simulink library "HndDriveReq"  (R2022a)
settings: Solver=VariableStepAuto  StartTime=0.0  StopTime=10.0  RelTol=1e-3
settings Model: Creator=DELL  LastModifiedBy=DELL

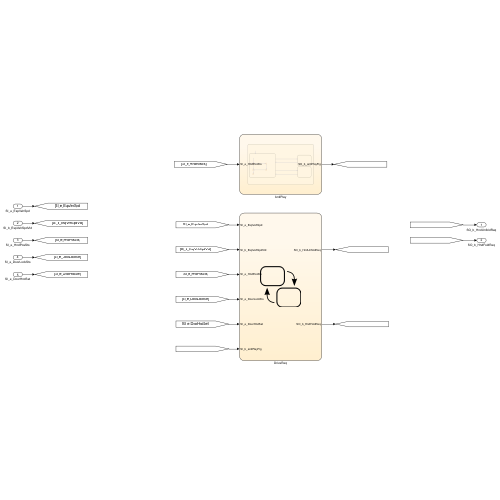
[thumbnail: Simulink's stored preview of the top-level diagram]
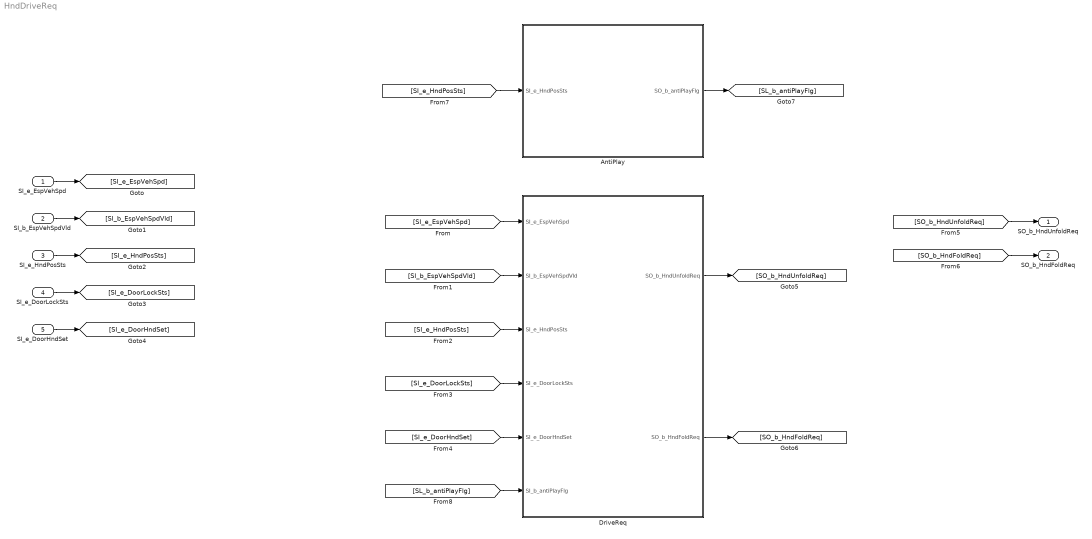
== system HndDriveReq ==
  SI_e_EspVehSpd : Inport
  SI_b_EspVehSpdVld : Inport  Port=2
  SI_e_HndPosSts : Inport  Port=3
  SI_e_DoorLockSts : Inport  Port=4
  SI_e_DoorHndSet : Inport  Port=5
  AntiPlay : Stateflow chart  TreatAsAtomicUnit=on
  DriveReq : Stateflow chart  TreatAsAtomicUnit=on
  SO_b_HndUnfoldReq : Outport
  SO_b_HndFoldReq : Outport  Port=2
  wires:
  SI_e_EspVehSpd/1 -> [SI_e_EspVehSpd]
  SI_b_EspVehSpdVld/1 -> [SI_b_EspVehSpdVld]
  SI_e_HndPosSts/1 -> [SI_e_HndPosSts]
  SI_e_DoorLockSts/1 -> [SI_e_DoorLockSts]
  SI_e_DoorHndSet/1 -> [SI_e_DoorHndSet]
  [SI_e_EspVehSpd] -> DriveReq/1(SI_e_EspVehSpd)
  [SI_b_EspVehSpdVld] -> DriveReq/2(SI_b_EspVehSpdVld)
  [SI_e_HndPosSts] -> DriveReq/3(SI_e_HndPosSts)
  [SI_e_DoorLockSts] -> DriveReq/4(SI_e_DoorLockSts)
  [SI_e_DoorHndSet] -> DriveReq/5(SI_e_DoorHndSet)
  [SO_b_HndUnfoldReq] -> SO_b_HndUnfoldReq/1
  [SO_b_HndFoldReq] -> SO_b_HndFoldReq/1
  DriveReq/1(SO_b_HndUnfoldReq) -> [SO_b_HndUnfoldReq]
  DriveReq/2(SO_b_HndFoldReq) -> [SO_b_HndFoldReq]
  [SI_e_HndPosSts] -> AntiPlay/1(SI_e_HndPosSts)
  AntiPlay/1(SO_b_antiPlayFlg) -> [SL_b_antiPlayFlg]
  [SL_b_antiPlayFlg] -> DriveReq/6(SI_b_antiPlayFlg)

== stateflow chart HndDriveReq/AntiPlay ==
  state AntiPlay
    state Count
      (default) -> (junction 4)
      Count -> (junction 4) [order 1]
      (junction 4) -> (junction 5) [order 1] : [hasChangedTo(SI_e_HndPosSts, 1) || ...
          | hasChangedTo(SI_e_HndPosSts, 0)]
      (junction 4) -> (junction 6) [order 2]
      (junction 5) -> (junction 7) : {SL_e_antiPlayCount ++}
      (junction 7) -> (junction 6)
      (junction 6) -> (junction 9)
    state TrigAndClean
      en:
      SO_b_antiPlayFlg = 1;
      SL_e_antiPlayCount = 0;
    state Clean
      en:
      SL_e_antiPlayCount = 0;
    (default) -> Count
    Count -> TrigAndClean [order 1] : [before(3000, tick) &&...
        | SL_e_antiPlayCount >= 10]
    TrigAndClean -> Count : after(18000, tick)
        | {SO_b_antiPlayFlg = 0;}
    Count -> Clean [order 2] : [after(3000, tick)]
    Clean -> Count
  data: SL_e_antiPlayCount local uint8 =0; SI_e_HndPosSts input uint8 =0; SO_b_antiPlayFlg output boolean =0

== stateflow chart HndDriveReq/DriveReq ==
  state Unfold [parallel]
    settings: executionOrder=1
    state Idle
      SO_b_HndUnfoldReq = 0;
    state NormalUnfoldReq
      en:
      SO_b_HndUnfoldReq = 1;
      on at(5, tick):
      SO_b_HndUnfoldReq = 0;
    state ExhibUnfoldReq
      en:
      SO_b_HndUnfoldReq = 1;
    state WashUnfoldReq
      en:
      SO_b_HndUnfoldReq = 1;
    (default) -> Unfold.Idle
    Unfold.Idle -> NormalUnfoldReq [order 1] : [((SI_e_EspVehSpd <= 20 && SI_b_EspVehSpdVld == 0) || ...
        | SI_b_EspVehSpdVld == 1) && ...
        | (SI_b_DoorAjar == 1 || SI_e_DoorLockSts == 1) && ...
        | SI_e_HndPosSts != 1]
    NormalUnfoldReq -> Unfold.Idle : [(SI_e_EspVehSpd > 20 && SI_b_EspVehSpdVld == 0) || ...
        | (SI_b_DoorAjar != 1 && SI_e_DoorLockSts != 1) || ...
        | SI_e_HndPosSts == 1]
        | {SO_b_HndUnfoldReq = 0;}
    Unfold.Idle -> ExhibUnfoldReq [order 2] : [hasChangedTo(SI_e_DoorHndSet, 4) && ...
        | SI_e_HndPosSts != 1]
    ExhibUnfoldReq -> Unfold.Idle : after(5, tick)
    Unfold.Idle -> WashUnfoldReq [order 3] : [hasChangedTo(SI_e_DoorHndSet, 3) && ...
        | SI_e_HndPosSts != 1]
    WashUnfoldReq -> Unfold.Idle : after(5, tick)
  state Fold [parallel]
    settings: executionOrder=2
    state Idle
      SO_b_HndFoldReq = 0;
    state FoldReq
      en:
      SO_b_HndFoldReq = 1;
    (default) -> Fold.Idle
    Fold.Idle -> FoldReq : [(SI_e_EspVehSpd > 20 && SI_b_EspVehSpdVld == 0) && ...
        | SI_e_DoorLockSts == 0 && ...
        | SL_b_antiPlayFlg == 0 && ...
        | SI_e_HndPosSts != 0]
    FoldReq -> Fold.Idle : [((SI_e_EspVehSpd <= 20 && SI_b_EspVehSpdVld == 0) || ...
        | SI_b_EspVehSpdVld == 1) || ...
        | SI_e_DoorLockSts != 0 || ...
        | SL_b_antiPlayFlg == 1 || ...
        | SI_e_HndPosSts == 0]
  data: SI_e_EspVehSpd input uint8; SI_b_EspVehSpdVld input boolean; SO_b_HndUnfoldReq output boolean; SL_e_antiPlayCount local uint8 =0; SI_e_HndPosSts input uint8; SI_e_DoorLockSts input uint8; SI_e_DoorHndSet input uint8; SO_b_HndFoldReq output boolean; SI_b_antiPlayFlg input boolean =0
